simulink model "test_4"  (R2024a)
settings: Solver=VariableStepAuto  StartTime=0.0  StopTime=1000  RelTol=1e-3
values from neighbouring files (symbols this model uses):
  A = zeros(6, 6)    [task4.m]    (also in task4_old.m)
  B = zeros(6,2)    [task4.m]    (also in task4_old.m)
  C = zeros(2,6)    [task4.m]    (also in task4_old.m)
  N = zeros(6,2)    [task4.m]    (also in task4_old.m; task6.m)
  R1 = diag([0.1,0.1])    [task4.m]    (also in task4_old.m = diag([10^-8,10^-8]); task6.m = diag([1e-15;1e-15]))
  R2 = 10^-10    (= 1e-10)    [task4.m]    (also in task4_old.m; task6.m)
libraries: simulink x1
settings Model: PacingRate=20  Creator=geopap-4  LastModifiedBy=geopap-4

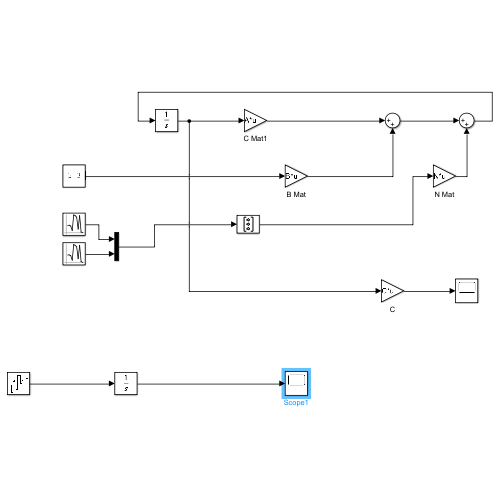
[thumbnail: Simulink's stored preview of the top-level diagram]
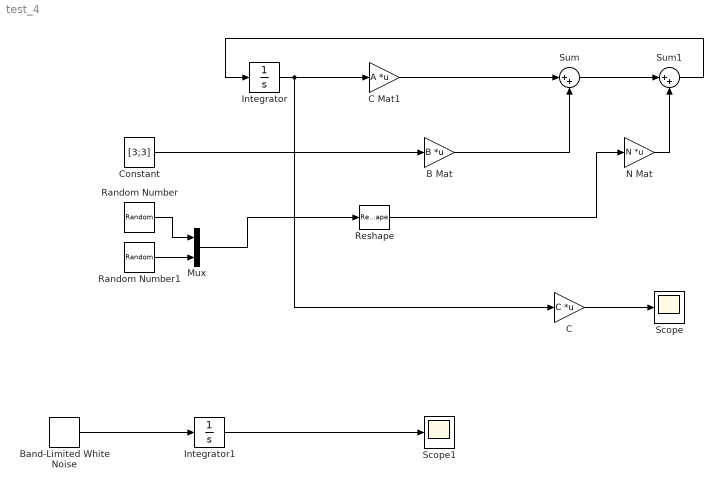
== system test_4 ==
  B Mat : Gain  Gain=B  Multiplication=Matrix(K*u)
  Band-Limited White Noise : simulink/Sources/Band-Limited White Noise  Cov=R1  Ts=0.1  seed=[23341]
  C : Gain  Gain=C  Multiplication=Matrix(K*u)
  C Mat1 : Gain  Gain=A  Multiplication=Matrix(K*u)
  Constant : Constant  Value=[3;3]
  Integrator : Integrator
  Integrator1 : Integrator
  Mux : Mux  Inputs=2
  N Mat : Gain  Gain=N  Multiplication=Matrix(K*u)
  Random Number : RandomNumber  Variance=R1  SampleTime=0.1
  Random Number1 : RandomNumber  Variance=R2  SampleTime=0.1
  Reshape : Reshape  OutputDimensionality=Column vector (2-D)
  Scope : Scope
  Scope1 : Scope
  Sum : Sum  Inputs=|++
  Sum1 : Sum  Inputs=|++
  wires:
  Integrator/1 -> C/1, C Mat1/1
  B Mat/1 -> Sum/2
  Constant/1 -> B Mat/1
  C Mat1/1 -> Sum/1
  Sum/1 -> Sum1/1
  N Mat/1 -> Sum1/2
  Mux/1 -> Reshape/1
  Random Number/1 -> Mux/1
  Random Number1/1 -> Mux/2
  Sum1/1 -> Integrator/1
  Reshape/1 -> N Mat/1
  C/1 -> Scope/1
  Band-Limited White Noise/1 -> Integrator1/1
  Integrator1/1 -> Scope1/1
